simulink model "InvPendulum"  (R2016b)
settings: Solver=ode4  StartTime=0.0  StopTime=0.5  FixedStep=0.01  RelTol=1e-3
undefined symbols (not defined in the file or in its folder): rhos
settings Model: Creator=Ernie  LastModifiedBy=Ernie
settings DebuggingCC: AlgebraicLoopMsg=none

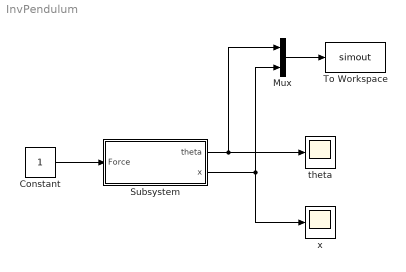
== system InvPendulum ==
  Constant : Constant
  Mux : Mux  Inputs=2
  Subsystem : Subsystem
  To Workspace : ToWorkspace  VariableName=simout  SaveFormat=Timeseries  SampleTime=-1
  theta : Scope
  x : Scope
  wires:
  Constant/1 -> Subsystem/1(Force)
  Subsystem/1(theta) -> Mux/1, theta/1
  Subsystem/2(x) -> Mux/2, x/1
  Mux/1 -> To Workspace/1

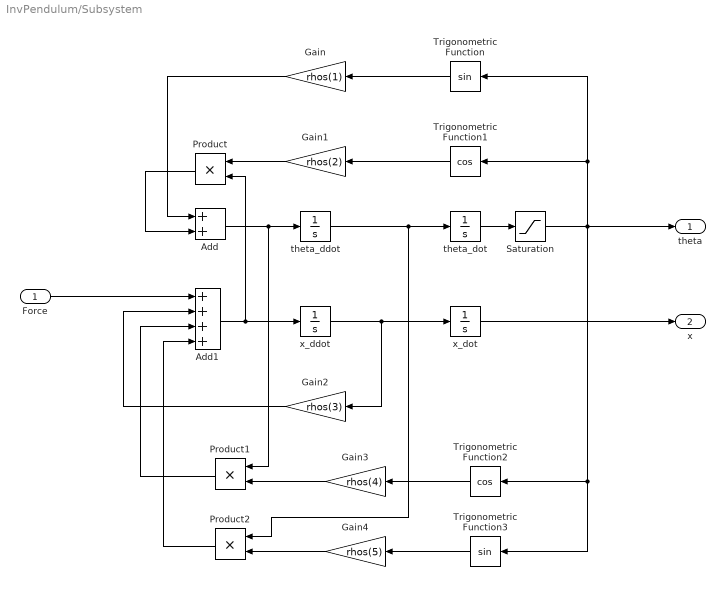
== system InvPendulum/Subsystem ==
  Force : Inport
  Add : Sum
  Add1 : Sum  Inputs=++++
  Gain : Gain  Gain=rhos(1)
  Gain1 : Gain  Gain=rhos(2)
  Gain2 : Gain  Gain=rhos(3)
  Gain3 : Gain  Gain=rhos(4)
  Gain4 : Gain  Gain=rhos(5)
  Product : Product
  Product1 : Product
  Product2 : Product
  Saturation : Saturate  UpperLimit=pi/2  LowerLimit=-pi/2
  Trigonometric Function : Trigonometry
  Trigonometric Function1 : Trigonometry  Operator=cos
  Trigonometric Function2 : Trigonometry  Operator=cos
  Trigonometric Function3 : Trigonometry
  theta_ddot : Integrator
  theta_dot : Integrator
  x_ddot : Integrator
  x_dot : Integrator
  theta : Outport
  x : Outport  Port=2
  wires:
  theta_ddot/1 -> Product2/1, theta_dot/1
  x_ddot/1 -> x_dot/1, Gain2/1
  x_dot/1 -> x/1
  Add1/1 -> x_ddot/1, Product/2
  Add/1 -> Product1/1, theta_ddot/1
  Trigonometric Function/1 -> Gain/1
  Gain/1 -> Add/1
  Force/1 -> Add1/1
  Trigonometric Function1/1 -> Gain1/1
  Gain1/1 -> Product/1
  Product/1 -> Add/2
  Gain2/1 -> Add1/2
  Trigonometric Function2/1 -> Gain3/1
  Gain3/1 -> Product1/2
  Product1/1 -> Add1/3
  Trigonometric Function3/1 -> Gain4/1
  Gain4/1 -> Product2/2
  Product2/1 -> Add1/4
  theta_dot/1 -> Saturation/1
  Saturation/1 -> Trigonometric Function3/1, Trigonometric Function2/1, Trigonometric Function1/1, Trigonometric Function/1, theta/1
